simulink subsystem "motortorquecmd"  (R2022b)
settings: Solver=VariableStepAuto  StartTime=0.0  StopTime=10.0  RelTol=1e-3
settings Model: Creator=serga  LastModifiedBy=serga

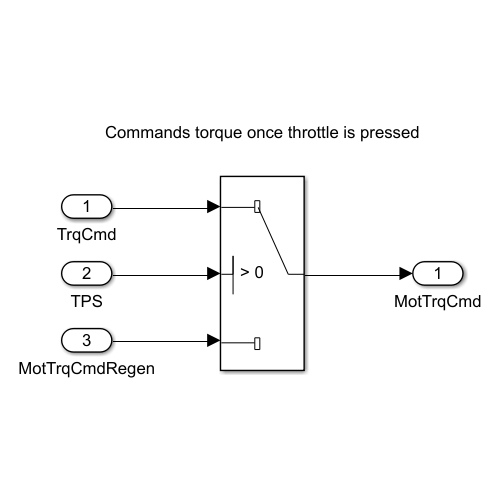
[thumbnail: Simulink's stored preview of the top-level diagram]
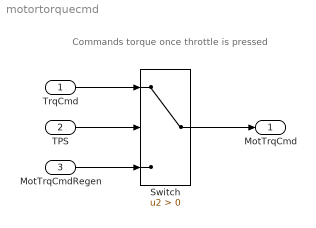
== system motortorquecmd ==
  note: Commands torque once throttle is pressed
  TrqCmd : Inport
  TPS : Inport  Port=2
  MotTrqCmdRegen : Inport  Port=3
  Switch : Switch  Criteria=u2 > Threshold  SaturateOnIntegerOverflow=off  InputSameDT=off
  MotTrqCmd : Outport
  wires:
  TPS/1 -> Switch/2
  TrqCmd/1 -> Switch/1
  MotTrqCmdRegen/1 -> Switch/3
  Switch/1 -> MotTrqCmd/1
